simulink model "ECEN315_PID"  (R2021a)
settings: Solver=FixedStepAuto  StartTime=0.0  StopTime=Inf  RelTol=1e-3  EnableMultiTasking=on
libraries: arduinolib x2
settings Model: SILPILModeSetting=veronly  ExtModeTrigDuration=2  Creator=zhuangxiao  LastModifiedBy=zhuangxiaobin
settings SolverCC: AlgebraicLoopSolver=TrustRegion
settings OptimizationCC: EnhancedBackFolding=on  PassReuseOutputArgsAs=Individual arguments  ZeroExternalMemoryAtStartup=off  ZeroInternalMemoryAtStartup=off  MaxStackSize=64  OptimizeBlockOrder=speed  DifferentSizesBufferReuse=on  OptimizationCustomize=off  EfficientTunableParamExpr=on
settings DebuggingCC: ParameterTunabilityLossMsg=error  SFMachineParentedDataDiag=warning
settings HardwareCC: ProdBitPerInt=16  ProdBitPerPointer=16  ProdBitPerSizeT=16  ProdBitPerPtrDiffT=16  ProdLargestAtomicFloat=None  ProdWordSize=8  ProdHWDeviceType=Atmel->AVR
settings SFSimCC: MATLABDynamicMemAlloc=off
settings RTWCC: SystemTargetFile=ert.tlc  HardwareBoard=Arduino Mega 2560  TemplateMakefile=ert_default_tmf  GenerateReport=on  Toolchain=Arduino AVR  BuildConfiguration=Faster Runs  IncludeHyperlinkInReport=on  LaunchReport=on  GenerateTraceInfo=on  GenerateTraceReport=on  GenerateTraceReportSl=on  GenerateTraceReportSf=on  GenerateTraceReportEml=on
settings CodeAppCC: ForceParamTrailComments=on  IgnoreCustomStorageClasses=off  OperatorAnnotations=on  SimulinkDataObjDesc=on  SFDataObjDesc=on  InsertBlockDesc=on
settings ERTTargetCC: SupportContinuousTime=on  SupportVariableSizeSignals=on  ExtModeStaticAllocSize=2048

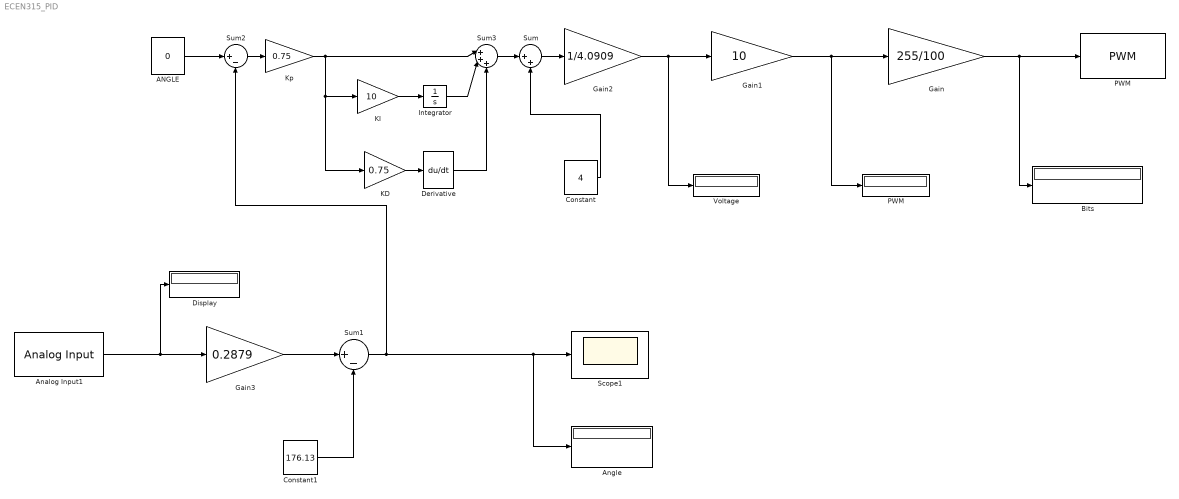
== system ECEN315_PID ==
  " KI " : Gain  Gain=10
  "ANGLE " : Constant  Value=0
  Analog Input1 : arduinolib/Analog Input  pinNumber=15  ReadResultsOnly=off  ConversionTriggerSource=Software  ExternalTriggerType=uint32(0)  OutputDataType=uint16  EnableConversionCompleteNotify=off  EnableOuputStatus=off  SampleTime=0.01  blockPlatform=arduino
  Angle : Display
  "Bits " : Display
  Constant : Constant  Value=4
  Constant1 : Constant  Value=176.13
  Derivative : Derivative
  Display : Display
  Gain : Gain  Gain=255/100
  Gain1 : Gain  Gain=10
  Gain2 : Gain  Gain=1/4.0909
  Gain3 : Gain  Gain=0.2879
  Integrator : Integrator  LimitOutput=on  LowerSaturationLimit=0
  KD : Gain  Gain=0.75
  Kp : Gain  Gain=0.75
  PWM : arduinolib/PWM  pinNumber=4  frequencyType=Default  desiredFrequency=490.2  achievableFrequency=490.2
  "PWM " : Display
  Scope1 : Scope
  Sum : Sum  Inputs=|++
  Sum1 : Sum  Inputs=|+-
  Sum2 : Sum  Inputs=|+-
  Sum3 : Sum  Inputs=|+++
  "Voltage " : Display
  wires:
  Gain/1 -> PWM/1, "Bits "/1
  Gain1/1 -> "PWM "/1, Gain/1
  Gain2/1 -> Gain1/1, "Voltage "/1
  Sum/1 -> Gain2/1
  Constant/1 -> Sum/2
  Constant1/1 -> Sum1/2
  Analog Input1/1 -> Gain3/1, Display/1
  Sum1/1 -> Angle/1, Scope1/1, Sum2/2
  "ANGLE "/1 -> Sum2/1
  Gain3/1 -> Sum1/1
  Sum3/1 -> Sum/1
  Sum2/1 -> Kp/1
  " KI "/1 -> Integrator/1
  Kp/1 -> KD/1, " KI "/1, Sum3/1
  Integrator/1 -> Sum3/2
  KD/1 -> Derivative/1
  Derivative/1 -> Sum3/3
